simulink model "Mcl_Floating_Signal_Processing"  (R2018a)
settings: Solver=VariableStepAuto  StartTime=0.0  StopTime=10.0  RelTol=1e-3
libraries: mciapi_libbrowser x4
settings Model: Creator=lab.motori2  LastModifiedBy=lab.motori2

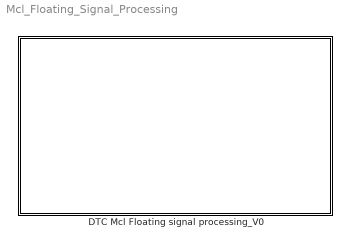
== system Mcl_Floating_Signal_Processing ==
  DTC Mcl Floating signal processing_V0 : Subsystem

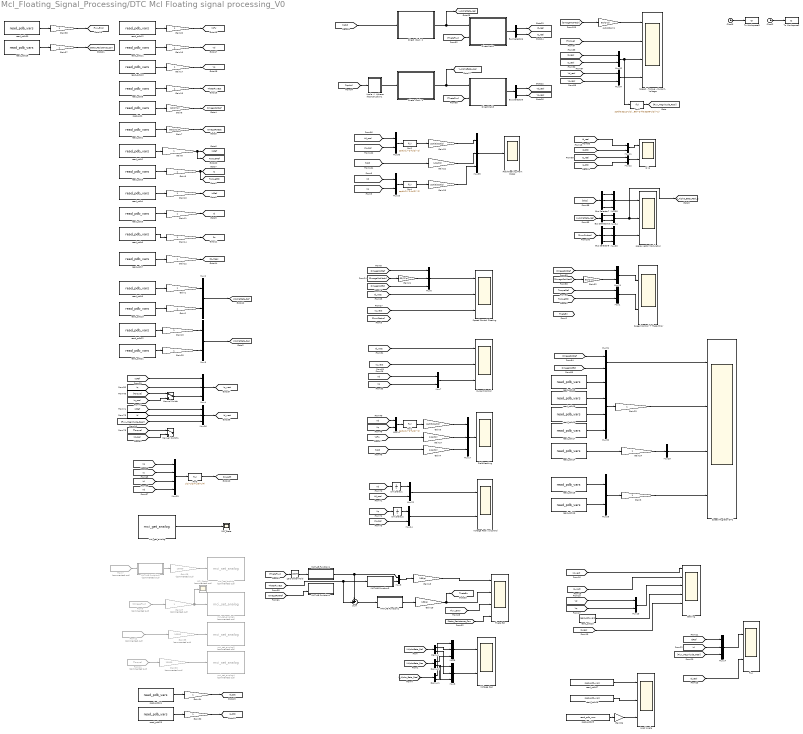
== system Mcl_Floating_Signal_Processing/DTC Mcl Floating signal processing_V0 ==
  Braking : Scope  NumInputPorts=6
  Bus Selector10 : BusSelector  OutputSignals=Alpha,Beta
  Bus Selector6 : BusSelector  OutputSignals=D,Q
  Bus Selector7 : BusSelector  OutputSignals=Ia,Ib,Ic
  Bus Selector8 : BusSelector  OutputSignals=A,B,C
  Bus Selector9 : BusSelector  OutputSignals=D,Q
  Clock2 : Clock
  Clock3 : Clock
  Current Control : Scope  NumInputPorts=3
  Demux : Demux  Outputs=2
  Demux1 : Demux  Outputs=2
  Demux2 : Demux  Outputs=2
  Direct  Clark  2 : MATLAB Function  TreatAsAtomicUnit=on  SystemSampleTime=SystemSampleTime  mask{SystemSampleTime=-1}
      mask prompts: SystemSampleTime "Simulink:blkprm_prompts:AllBlksSampleTime"
  Direct  Clark  3 : MATLAB Function  TreatAsAtomicUnit=on  SystemSampleTime=SystemSampleTime  mask{SystemSampleTime=-1}
      mask prompts: SystemSampleTime "Simulink:blkprm_prompts:AllBlksSampleTime"
  Direct Park2 : MATLAB Function  TreatAsAtomicUnit=on  SystemSampleTime=SystemSampleTime  mask{SystemSampleTime=-1}
      mask prompts: SystemSampleTime "Simulink:blkprm_prompts:AllBlksSampleTime"
  Direct Park3 : MATLAB Function  TreatAsAtomicUnit=on  SystemSampleTime=SystemSampleTime  mask{SystemSampleTime=-1}
      mask prompts: SystemSampleTime "Simulink:blkprm_prompts:AllBlksSampleTime"
  Fcn1 : Fcn  Expr=sqrt(u(1)^2+u(2)^2)
  Fcn2 : Fcn  Expr=sqrt(u(1)^2+u(2)^2)
  Fcn3 : Fcn  Expr=u(1)*u(2)+u(3)*u(4)
  Fcn4 : Fcn  Expr=sqrt(u(1)^2+u(2)^2)
  Fcn5 : Fcn  Expr=sqrt((0.0212*u(1)+0.0688)^2+(0.0299*u(2))^2)
  "FieldWeaking " : Scope
  FieldWeaking From Model : Scope
  Flux : Scope  NumInputPorts=2
  From11 : From  Commented=on  GotoTag=Torque  TagVisibility=global
  From12 : From  Commented=on  GotoTag=Flux_Magnitude_Real
  From7 : From  Commented=on  GotoTag=Stator_Flux_Position_Real
  From9 : From  Commented=on  GotoTag=OmegaFlux  TagVisibility=global
  Gain{1..3,8..17,20,23..25,30,34,37..38} (21 alike) : Gain  OutDataTypeStr=double  RndMeth=Zero
  Gain18 : Gain  Gain=180/pi
  Gain19 : Gain  Gain=180/pi
  Gain21 : Gain  Gain=60/(2*pi)  RndMeth=Round
  Gain22 : Gain  Gain=1/sqrt(2)
  Gain26 : Gain  Gain=sqrt(3)/sqrt(2)
  Gain27 : Gain  Gain=1/sqrt(2)
  Gain28 : Gain  Commented=on  Gain=10000  OutDataTypeStr=int32
  Gain29 : Gain  Commented=on  OutDataTypeStr=int32
  Gain31 : Gain  Gain=sqrt(3)/sqrt(2)
  Gain32 : Gain  Gain=60/(2*pi)  RndMeth=Round
  Gain33 : Gain  Commented=on  Gain=10000  OutDataTypeStr=int32
  Gain35 : Gain  Commented=on  Gain=10000  OutDataTypeStr=int32
  Gain36 : Gain  Gain=180/pi
  Gain4 : Gain  Gain=1/sqrt(2)
  Gain5 : Gain  Gain=sqrt(3)/sqrt(2)
  Gain6 : Gain  Gain=60/(2*pi)  OutDataTypeStr=double  RndMeth=Zero
  Gain7 : Gain  Gain=60/(2*pi)/4  OutDataTypeStr=double  RndMeth=Zero
  Id iq : Scope  NumInputPorts=2
  Load Angle : Scope  NumInputPorts=3
  MATLAB Function1 : MATLAB Function  TreatAsAtomicUnit=on
  MATLAB Function2 : MATLAB Function  TreatAsAtomicUnit=on
  MATLAB Function3 : MATLAB Function  TreatAsAtomicUnit=on
  MATLAB Function4 : MATLAB Function  TreatAsAtomicUnit=on
  MATLAB Function5 : MATLAB Function  Commented=on  TreatAsAtomicUnit=on
  MCI_State : Scope
  MCI_State1 : Scope  Commented=on
  Manual Switch : ManualSwitch
  Manual Switch1 : ManualSwitch
  Mux{1..3,7,9..13,18,21..22,24,28,31..32,34,36..37} (19 alike) : Mux  Inputs=2
  Mux{4..6,8,14,17,26,33,35,38} (10 alike) : Mux  Inputs=3
  Mux23 : Mux
  Mux29 : Mux  Inputs=1
  Mux30 : Mux
  Speed - Torque - Current - Voltage : Scope  NumInputPorts=4
  Speed Control + Theta Error : Scope  NumInputPorts=2
  "Speed Control Floating " : Scope  NumInputPorts=3
  "Speed Ruglator DTC " : Scope  NumInputPorts=4
  Sum : Sum  Inputs=+-|
  Theta Est : Scope  NumInputPorts=4
  To Workspace2 : ToWorkspace  VariableName=t2  SampleTime=-1
      settings: Save2DSignal=2-D array (concatenate along first dimension)
  To Workspace3 : ToWorkspace  VariableName=t3  SampleTime=-1
      settings: Save2DSignal=2-D array (concatenate along first dimension)
  Unit Delay1 : UnitDelay  SampleTime=-1
  Unit Delay2 : UnitDelay  SampleTime=-1
  Voltage Real vs Control : Scope  NumInputPorts=2
  Voltage Rec : Scope  NumInputPorts=2
  "Vpole -> Vphase reconstruction1" : MATLAB Function  TreatAsAtomicUnit=on
  Zero-Order Hold : ZeroOrderHold  SampleTime=0.000125
  mci_get_analog : S-Function  FunctionName=mci_get_analog  Parameters=read_data, choose_read_data  SFunctionDeploymentMode=off  EnableBusSupport=off  mask{choose_read_data=MCI_AI_INTERNAL_MCI_STATE, read_data=24}
      mask prompts: choose_read_data "Data to read"
      mask TypeOptions choose_read_data: MCI_AI_TARGET_SPEED_RPM_S16 | MCI_AI_SPEED_REFERENCE_RPM_S16 | MCI_AI_ACTUAL_SPEED_S16 | MCI_AI_SPEED_ERROR_RPM_S16 | MCI_AI_MEAN_SPEED_S16 | MCI_AI_RMS_MOTOR_CURRENT_S16 | MCI_AI_ACTIVE_POWER_S16 | MCI_AI_SHAFT_POWER_S16 | MCI_AI_MOTOR_TEMP_S16 | MCI_AI_STATOR_TEMP_S16 | MCI_AI_LOAD_TORQUE_S16 | MCI_AI_SHAFT_POSITION_DEG_S16 | MCI_AI_BUS_CURRENT_S16 | MCI_AI_BUS_VOLTAGE_S16 | MCI_AI_INVERTER_TEMP_S16 | MCI_AI_INVERTER_TEMP_RAW_DATA | MCI_AI_VOLTAGE_PHASE_A_S16 | MCI_AI_VOLTAGE_PHASE_B_S16 | MCI_AI_VOLTAGE_PHASE_C_S16 | MCI_AI_SPEED_LOOP_GAIN_TABLE_INDEX | MCI_AI_CURR_PHASE_A_S16 | MCI_AI_CURR_PHASE_B_S16 | MCI_AI_CURR_PHASE_C_S16 | MCI_AI_STATOR_RESISTANCE_S16 | MCI_AI_INTERNAL_MCI_STATE
      mask Callback read_data:
      | rd = get_param(gcb,'choose_read_data');
      | poenum = strcat('MCI_AI_TYPE.',rd);
      | i_32 = eval(['int32(' poenum ')']);
      | set_param(gcb,'read_data',int2str(i_32));
      mask Display:
      | disp = regexp(choose_read_data, 'MCI_AI_', 'split');
      | port_label('output', 1, disp{2});
  mci_set_analog : mciapi_libbrowser/mci_set_analog  Commented=on  choose_write_data=MCI_AO_SPEED_LOOP_PROP_GAIN_S16  write_data=0
      settings: SourceProductName=Sim Arch
  mci_set_analog1 : mciapi_libbrowser/mci_set_analog  Commented=on  choose_write_data=MCI_AO_SPEED_LOOP_INT_GAIN_S16  write_data=1
      settings: SourceProductName=Sim Arch
  mci_set_analog3 : mciapi_libbrowser/mci_set_analog  Commented=on  choose_write_data=MCI_AO_SOFTSTART_COUNTER_INDEX  write_data=4
      settings: SourceProductName=Sim Arch
  mci_set_analog4 : mciapi_libbrowser/mci_set_analog  Commented=on  choose_write_data=MCI_AO_SPEED_FIR_TAPS_TABLE_INDEX  write_data=3
      settings: SourceProductName=Sim Arch
  rad/s2Rpm1 : Gain  Gain=60/(2*pi)
  read_pdb : S-Function  FunctionName=read_pdb_vars  Parameters=vstring  SFunctionDeploymentMode=off  EnableBusSupport=off  mask{vstring=Mcl_IO.Speed_Rot_Ref}
      mask prompts: vstring "Variable to read"
      mask Display:
      | disp = vstring;
      | port_label('output', 1, disp);
  read_pdb1 : S-Function  FunctionName=read_pdb_vars  Parameters=vstring  SFunctionDeploymentMode=off  EnableBusSupport=off  mask{vstring=Mcl_Quantities.Speed_Rot}
      mask prompts: vstring "Variable to read"
      mask Display:
      | disp = vstring;
      | port_label('output', 1, disp);
  read_pdb10 : S-Function  FunctionName=read_pdb_vars  Parameters=vstring  SFunctionDeploymentMode=off  EnableBusSupport=off  mask{vstring=Mcl_Quantities.Vs_DQ.Q}
      mask prompts: vstring "Variable to read"
      mask Display:
      | disp = vstring;
      | port_label('output', 1, disp);
  read_pdb11 : S-Function  FunctionName=read_pdb_vars  Parameters=vstring  SFunctionDeploymentMode=off  EnableBusSupport=off  mask{vstring=Mcl_Quantities.Vs_DQ.D}
      mask prompts: vstring "Variable to read"
      mask Display:
      | disp = vstring;
      | port_label('output', 1, disp);
  read_pdb12 : S-Function  FunctionName=read_pdb_vars  Parameters=vstring  SFunctionDeploymentMode=off  EnableBusSupport=off  mask{vstring=Mcl_Quantities.Vs_Max_Filt}
      mask prompts: vstring "Variable to read"
      mask Display:
      | disp = vstring;
      | port_label('output', 1, disp);
  read_pdb13 : S-Function  FunctionName=read_pdb_vars  Parameters=vstring  SFunctionDeploymentMode=off  EnableBusSupport=off  mask{vstring=Speed_Controller.Upper_Limit}
      mask prompts: vstring "Variable to read"
      mask Display:
      | disp = vstring;
      | port_label('output', 1, disp);
  read_pdb14 : S-Function  FunctionName=read_pdb_vars  Parameters=vstring  SFunctionDeploymentMode=off  EnableBusSupport=off  mask{vstring=Load_Angle_Limiter.Err}
      mask prompts: vstring "Variable to read"
      mask Display:
      | disp = vstring;
      | port_label('output', 1, disp);
  read_pdb15 : S-Function  FunctionName=read_pdb_vars  Parameters=vstring  SFunctionDeploymentMode=off  EnableBusSupport=off  mask{vstring=Load_Angle_Limiter.Upper_Limit}
      mask prompts: vstring "Variable to read"
      mask Display:
      | disp = vstring;
      | port_label('output', 1, disp);
  read_pdb16 : S-Function  FunctionName=read_pdb_vars  Parameters=vstring  SFunctionDeploymentMode=off  EnableBusSupport=off  mask{vstring=Load_Angle_Limiter.Out}
      mask prompts: vstring "Variable to read"
      mask Display:
      | disp = vstring;
      | port_label('output', 1, disp);
  read_pdb17 : S-Function  FunctionName=read_pdb_vars  Parameters=vstring  SFunctionDeploymentMode=off  EnableBusSupport=off  mask{vstring=Speed_Controller.Lower_Limit}
      mask prompts: vstring "Variable to read"
      mask Display:
      | disp = vstring;
      | port_label('output', 1, disp);
  read_pdb18 : S-Function  FunctionName=read_pdb_vars  Parameters=vstring  SFunctionDeploymentMode=off  EnableBusSupport=off  mask{vstring=Speed_Controller.Out}
      mask prompts: vstring "Variable to read"
      mask Display:
      | disp = vstring;
      | port_label('output', 1, disp);
  read_pdb19 : S-Function  FunctionName=read_pdb_vars  Parameters=vstring  SFunctionDeploymentMode=off  EnableBusSupport=off  mask{vstring=Mcl_Quantities.Vs_Alpha_Beta.Beta}
      mask prompts: vstring "Variable to read"
      mask Display:
      | disp = vstring;
      | port_label('output', 1, disp);
  read_pdb2 : S-Function  FunctionName=read_pdb_vars  Parameters=vstring  SFunctionDeploymentMode=off  EnableBusSupport=off  mask{vstring=Mcl_Quantities.Torque_Ref}
      mask prompts: vstring "Variable to read"
      mask Display:
      | disp = vstring;
      | port_label('output', 1, disp);
  read_pdb20 : S-Function  FunctionName=read_pdb_vars  Parameters=vstring  SFunctionDeploymentMode=off  EnableBusSupport=off  mask{vstring=Mcl_Quantities.Torque_Ref}
      mask prompts: vstring "Variable to read"
      mask Display:
      | disp = vstring;
      | port_label('output', 1, disp);
  read_pdb21 : S-Function  FunctionName=read_pdb_vars  Parameters=vstring  SFunctionDeploymentMode=off  EnableBusSupport=off  mask{vstring=Mcl_Quantities.Vs_Alpha_Beta_Rec.Beta}
      mask prompts: vstring "Variable to read"
      mask Display:
      | disp = vstring;
      | port_label('output', 1, disp);
  read_pdb22 : S-Function  FunctionName=read_pdb_vars  Parameters=vstring  SFunctionDeploymentMode=off  EnableBusSupport=off  mask{vstring=Mcl_Quantities.Vs_Alpha_Beta_Rec.Alpha}
      mask prompts: vstring "Variable to read"
      mask Display:
      | disp = vstring;
      | port_label('output', 1, disp);
  read_pdb23 : S-Function  FunctionName=read_pdb_vars  Parameters=vstring  SFunctionDeploymentMode=off  EnableBusSupport=off  mask{vstring=rotor_curr_iq}
      mask prompts: vstring "Variable to read"
      mask Display:
      | disp = vstring;
      | port_label('output', 1, disp);
  read_pdb24 : S-Function  FunctionName=read_pdb_vars  Parameters=vstring  SFunctionDeploymentMode=off  EnableBusSupport=off  mask{vstring=rotor_curr_id}
      mask prompts: vstring "Variable to read"
      mask Display:
      | disp = vstring;
      | port_label('output', 1, disp);
  read_pdb25 : S-Function  FunctionName=read_pdb_vars  Parameters=vstring  SFunctionDeploymentMode=off  EnableBusSupport=off  mask{vstring=Id_Braking}
      mask prompts: vstring "Variable to read"
      mask Display:
      | disp = vstring;
      | port_label('output', 1, disp);
  read_pdb26 : S-Function  FunctionName=read_pdb_vars  Parameters=vstring  SFunctionDeploymentMode=off  EnableBusSupport=off  mask{vstring=Stator_Resistance_Corr}
      mask prompts: vstring "Variable to read"
      mask Display:
      | disp = vstring;
      | port_label('output', 1, disp);
  read_pdb27 : S-Function  FunctionName=read_pdb_vars  Parameters=vstring  SFunctionDeploymentMode=off  EnableBusSupport=off  mask{vstring=Mcl_Quantities.Load_Angle_Sin_Cos.Sin}
      mask prompts: vstring "Variable to read"
      mask Display:
      | disp = vstring;
      | port_label('output', 1, disp);
  read_pdb28 : S-Function  FunctionName=read_pdb_vars  Parameters=vstring  SFunctionDeploymentMode=off  EnableBusSupport=off  mask{vstring=Mcl_Quantities.Load_Angle_Sin_Cos.Cos}
      mask prompts: vstring "Variable to read"
      mask Display:
      | disp = vstring;
      | port_label('output', 1, disp);
  read_pdb29 : S-Function  FunctionName=read_pdb_vars  Parameters=vstring  SFunctionDeploymentMode=off  EnableBusSupport=off  mask{vstring=Mcl_Quantities.Load_Angle}
      mask prompts: vstring "Variable to read"
      mask Display:
      | disp = vstring;
      | port_label('output', 1, disp);
  read_pdb3 : S-Function  FunctionName=read_pdb_vars  Parameters=vstring  SFunctionDeploymentMode=off  EnableBusSupport=off  mask{vstring=Mcl_Quantities.Torque}
      mask prompts: vstring "Variable to read"
      mask Display:
      | disp = vstring;
      | port_label('output', 1, disp);
  read_pdb30 : S-Function  FunctionName=read_pdb_vars  Parameters=vstring  SFunctionDeploymentMode=off  EnableBusSupport=off  mask{vstring=Flux_Error}
      mask prompts: vstring "Variable to read"
      mask Display:
      | disp = vstring;
      | port_label('output', 1, disp);
  read_pdb4 : S-Function  FunctionName=read_pdb_vars  Parameters=vstring  SFunctionDeploymentMode=off  EnableBusSupport=off  mask{vstring=Mcl_Quantities.Flux_Ref}
      mask prompts: vstring "Variable to read"
      mask Display:
      | disp = vstring;
      | port_label('output', 1, disp);
  read_pdb5 : S-Function  FunctionName=read_pdb_vars  Parameters=vstring  SFunctionDeploymentMode=off  EnableBusSupport=off  mask{vstring=Mcl_Quantities.Stator_Flux_Mag}
      mask prompts: vstring "Variable to read"
      mask Display:
      | disp = vstring;
      | port_label('output', 1, disp);
  read_pdb6 : S-Function  FunctionName=read_pdb_vars  Parameters=vstring  SFunctionDeploymentMode=off  EnableBusSupport=off  mask{vstring=Mcl_Quantities.Stator_Resistance}
      mask prompts: vstring "Variable to read"
      mask Display:
      | disp = vstring;
      | port_label('output', 1, disp);
  read_pdb7 : S-Function  FunctionName=read_pdb_vars  Parameters=vstring  SFunctionDeploymentMode=off  EnableBusSupport=off  mask{vstring=Estimated_Resistance}
      mask prompts: vstring "Variable to read"
      mask Display:
      | disp = vstring;
      | port_label('output', 1, disp);
  read_pdb8 : S-Function  FunctionName=read_pdb_vars  Parameters=vstring  SFunctionDeploymentMode=off  EnableBusSupport=off  mask{vstring=Mcl_Quantities.Rotor_Position}
      mask prompts: vstring "Variable to read"
      mask Display:
      | disp = vstring;
      | port_label('output', 1, disp);
  read_pdb9 : S-Function  FunctionName=read_pdb_vars  Parameters=vstring  SFunctionDeploymentMode=off  EnableBusSupport=off  mask{vstring=Mcl_Quantities.Vs_Alpha_Beta.Alpha}
      mask prompts: vstring "Variable to read"
      mask Display:
      | disp = vstring;
      | port_label('output', 1, disp);
  space vector Modulation : Scope  NumInputPorts=3
  tag scope: Flux_Error=global, I_AlphaBeta_real=global, Id=global, IdRef=global, Id_Est=global, Id_real=global, Id_vect=global, Iq=global, IqRef=global, Iq_Est=global, Iq_real=global, Iq_vect=global, OmegaRotEst=global, OmegaRotRef=global, PowerEl=global, Rs=global, Rs_Meas=global, Stator_Resistance_Corr=global, ThetaErr=global, ThetaFluxEst=global, TorqueEst=global, TorqueRef=global, VAlphaBeta_Rec=global, VAlphaBeta_Ref=global, V_AlphaBeta_real=global, V_Alpha_Beta_Real_s=global, Vd=global, Vd_real=global, Vq=global, Vq_real=global, VsFw=global
  wires:
  [OmegaRotMech] -> Gain21/1
  Mux6/1 -> "Speed Control Floating "/1  "Speed Reference - Real - Estimated"
  [OmegaRotRef] -> Mux6/1
  [Id_vect] -> "Speed Control Floating "/2  "D Reference [Current on FOC - Flux on DTC]"
  Mux7/1 -> Current Control/3  "Vdq"
  [Vd] -> Mux7/1
  [Vq] -> Mux7/2
  [ThetaFlux] -> Zero-Order Hold/1
  Mux9/1 -> Gain18/1
  MATLAB Function1/1(Theta_out) -> Sum/1, Mux9/1
  Gain18/1 -> Theta Est/1  "Theta Flux Vs Theta Est"
  Sum/1 -> MATLAB Function2/1(Theta_in)
  Gain19/1 -> [ThetaErr], Theta Est/2  "Theta Err [deg]"
  MATLAB Function2/1(Theta_out) -> Gain19/1
  Fcn1/1 -> Gain5/1
  Mux18/1 -> Fcn1/1
  [Vd] -> Mux18/1
  [Vq] -> Mux18/2
  [VsFw] -> Gain27/1
  Mux17/1 -> "FieldWeaking "/1  "Vs Motor - VsLimit - Vdc"
  Gain27/1 -> Mux17/2  "Vs Limit"
  [Vdc] -> Gain4/1
  [OmegaRotRef] -> MATLAB Function4/2(omega_rot_ref)
  Mux22/1 -> Voltage Real vs Control/1  "Vd Control vs Vd Real"
  Mux24/1 -> Voltage Real vs Control/2  "Vq Control vs Vq Real"
  [Vd] -> Unit Delay1/1
  [Vq_real] -> Mux24/2
  [Vq] -> Unit Delay2/1
  [Vd_real] -> Mux22/2
  Unit Delay1/1 -> Mux22/1
  Unit Delay2/1 -> Mux24/1
  [Iq_vect] -> "Speed Control Floating "/3  "Q Reference [Current on FOC - Torque on DTC]"
  MATLAB Function3/1(Theta_out) -> Mux9/2
  Gain4/1 -> Mux17/3  "Vdc"
  Gain5/1 -> Mux17/1  "Vs_Motor"
  Zero-Order Hold/1 -> MATLAB Function1/1(Theta_in)
  [ThetaFluxEst] -> Sum/2, MATLAB Function3/1(Theta_in)
  Gain21/1 -> Mux6/2  "Speed Real"
  [OmegaRotEst] -> Mux6/3
  read_pdb15/1 -> Mux28/1
  Mux28/1 -> Gain3/1  "Load Angle"
  read_pdb16/1 -> Mux28/2
  Gain24/1 -> Mux29/1
  Mux29/1 -> "Speed Ruglator DTC "/3
  Mux31/1 -> "Speed Ruglator DTC "/1  "Speed"
  Mux30/1 -> Gain23/1
  Gain23/1 -> "Speed Ruglator DTC "/2  "Torque"
  read_pdb14/1 -> Gain24/1
  [OmegaRotRef] -> Mux31/1
  [OmegaRotEst] -> Mux31/2
  Mux36/1 -> Fcn2/1
  Fcn2/1 -> Gain31/1
  Bus Selector6/1 -> [Id_real]  "<D>"
  [Vpole] -> "Vpole -> Vphase reconstruction1"/1(Vpole)
  Mux38/1 -> space vector Modulation/1  "Current A B C"
  [Vq_real] -> Mux37/2  "Vq"
  Gain22/1 -> Mux35/2  "Vdc"
  Bus Selector6/2 -> [Iq_real]  "<Q>"
  Bus Selector7/2 -> Mux38/2  "<Ib>"
  [Vd_real] -> Mux36/1  "Vd_real"
  "Vpole -> Vphase reconstruction1"/1(Vout) -> Direct  Clark  3/1(Xabc)
  [Vq_real] -> Mux36/2  "Vq_real"
  [ThetaFlux] -> Direct Park3/2(Theta)
  Gain31/1 -> Mux35/1  "Vs_Motor"
  Mux32/1 -> Fcn5/1, Speed - Torque - Current - Voltage/3
  Direct Park2/1(Xdq) -> Bus Selector6/1
  Clock2/1 -> To Workspace2/1
  [Iq_real] -> Mux32/2  "Iq"
  rad/s2Rpm1/1 -> Speed - Torque - Current - Voltage/1  "Speed"
  [PwmDuties] -> Bus Selector8/1
  Bus Selector7/1 -> Mux38/1  "<Ia>"
  Bus Selector7/3 -> Mux38/3  "<Ic>"
  Mux37/1 -> Speed - Torque - Current - Voltage/4
  Clock3/1 -> To Workspace3/1
  [Iabc] -> Direct  Clark  2/1(Xabc)
  [Iabc] -> Bus Selector7/1
  Bus Selector9/1 -> [Vd_real]  "<D>"
  [ThetaFlux] -> Direct Park2/2(Theta)
  Bus Selector8/3 -> Mux33/3  "<C>"
  [Torque] -> Speed - Torque - Current - Voltage/2  "Torque"
  [Id_real] -> Mux32/1  "Id"
  Bus Selector10/1 -> Mux34/1  "<Alpha>"
  Mux33/1 -> space vector Modulation/3  "Pwm Duties"
  [Vd_real] -> Mux37/1  "Vd"
  Bus Selector9/2 -> [Vq_real]  "<Q>"
  Bus Selector10/2 -> Mux34/2  "<Beta>"
  Mux34/1 -> [V_Alpha_Beta_Real_s], space vector Modulation/2  "V Alpha Beta"
  Bus Selector8/1 -> Mux33/1  "<A>"
  Bus Selector8/2 -> Mux33/2  "<B>"
  [V_AlphaBeta_real] -> Bus Selector10/1
  Mux35/1 -> FieldWeaking From Model/1
  Direct  Clark  3/1(XAlphaBeta) -> Direct Park3/1(XAlphaBeta), [V_AlphaBeta_real]  "Valpha_Beta_reconstructed"
  [Vdc] -> Gain22/1  "Vdc"
  Direct Park3/1(Xdq) -> Bus Selector9/1
  Direct  Clark  2/1(XAlphaBeta) -> [I_AlphaBeta_real], Direct Park2/1(XAlphaBeta)
  [OmegaRotMech] -> rad/s2Rpm1/1
  Gain8/1 -> [TorqueRef], [IqRef]
  read_pdb4/1 -> Gain10/1
  Gain11/1 -> [Id]
  Gain9/1 -> [TorqueEst], [Iq]
  read_pdb/1 -> Gain6/1
  Gain14/1 -> [Rs]
  read_pdb10/1 -> Gain17/1
  Gain20/1 -> [VsFw]
  read_pdb7/1 -> Gain12/1
  Gain12/1 -> [Rs_Meas]
  read_pdb8/1 -> Gain15/1
  Gain15/1 -> [ThetaFluxEst]
  Gain17/1 -> [Vq]  "Vq"
  Gain10/1 -> [IdRef]
  read_pdb3/1 -> Gain9/1
  read_pdb5/1 -> Gain11/1
  read_pdb2/1 -> Gain8/1
  read_pdb12/1 -> Gain20/1
  Gain6/1 -> [OmegaRotRef]
  read_pdb1/1 -> Gain7/1
  read_pdb6/1 -> Gain14/1
  Gain16/1 -> [Vd]  "Vd"
  read_pdb11/1 -> Gain16/1
  Gain7/1 -> [OmegaRotEst]
  read_pdb17/1 -> Mux30/4
  read_pdb20/1 -> Mux30/3
  read_pdb18/1 -> Mux30/2
  Gain3/1 -> "Speed Ruglator DTC "/4  "Load Angle"
  [Id_vect] -> Current Control/1  "D Reference [Current on FOC - Flux on DTC"
  [Iq_vect] -> Current Control/2  "Q Reference [Current on FOC - Torque on DTC]"
  [TorqueEst] -> Mux1/2
  [TorqueRef] -> Mux1/1
  Mux1/1 -> Speed Control + Theta Error/2  "Torque"
  [OmegaRotMech] -> Gain32/1
  Gain32/1 -> Mux21/2  "Motor Speed"
  [OmegaRotRef] -> Mux21/1  "Target Speed"
  Mux21/1 -> Speed Control + Theta Error/1
  read_pdb13/1 -> Mux30/1
  [Id] -> Mux26/2
  [Iq] -> Mux4/2
  [IqRef] -> Mux4/1
  [Torque] -> Manual Switch1/1
  [Iq_real] -> Manual Switch/2
  [Torque] -> Manual Switch/1
  Mux26/1 -> [Id_vect]  "Id"
  Manual Switch/1 -> Mux4/3
  [IdRef] -> Mux26/1
  [Vq] -> Mux23/1
  [Id_real] -> Manual Switch1/2
  Fcn3/1 -> [PowerEl]  "Power"
  mci_get_analog/1 -> MCI_State/1  "MCI_State"
  Mux23/1 -> Fcn3/1
  Mux4/1 -> [Iq_vect]  "Iq"
  [Vd] -> Mux23/4
  [Id] -> Mux23/3
  [Iq] -> Mux23/2
  read_pdb19/1 -> Gain2/1
  read_pdb9/1 -> Gain1/1
  Gain1/1 -> Mux2/1
  Gain2/1 -> Mux2/2
  Mux2/1 -> [VAlphaBeta_Ref]  "V Alpha Beta Ref"
  Mux3/1 -> [VAlphaBeta_Rec]  "V Alpha Beta Rec"
  read_pdb22/1 -> Gain13/1
  Gain13/1 -> Mux3/1
  Gain25/1 -> Mux3/2
  read_pdb21/1 -> Gain25/1
  [Vd] -> Mux10/1
  Mux10/1 -> Fcn4/1
  Fcn4/1 -> Gain26/1
  [Vq] -> Mux10/2
  Gain26/1 -> Mux35/3  "Vs Motor Ref"
  [VAlphaBeta_Ref] -> Demux/1
  Mux5/1 -> Voltage Rec/1  "VAlpha"
  Demux1/2 -> Mux8/1
  Demux1/1 -> Mux5/1
  [V_Alpha_Beta_Real_s] -> Demux1/1
  Mux8/1 -> Voltage Rec/2  "VBeta"
  Demux2/2 -> Mux8/3
  [VAlphaBeta_Rec] -> Demux2/1
  Demux/2 -> Mux8/2
  Demux/1 -> Mux5/2
  Demux2/1 -> Mux5/3
  From7/1 -> MATLAB Function5/1(Theta_in)
  From9/1 -> Gain29/1
  Gain28/1 -> mci_set_analog/1
  Gain29/1 -> MCI_State1/1, mci_set_analog1/1
  MATLAB Function5/1(Theta_out) -> Gain28/1
  Gain35/1 -> mci_set_analog3/1
  Gain33/1 -> mci_set_analog4/1
  From11/1 -> Gain33/1
  [Flux_Magnitude_Real] -> Mux26/3
  From12/1 -> Gain35/1
  read_pdb24/1 -> Gain34/1
  Gain34/1 -> [Id_Est]
  Gain30/1 -> [Iq_Est]
  read_pdb23/1 -> Gain30/1
  [Id_real] -> Mux11/1  "Id_rot"
  [Id_Est] -> Mux11/2
  Mux11/1 -> Id iq/1
  Mux12/1 -> Id iq/2
  [Iq_real] -> Mux12/1  "Iq_rot"
  [Iq_Est] -> Mux12/2
  Mux13/1 -> Braking/3  "Vdq"
  [Vd] -> Mux13/1
  [Vq] -> Mux13/2
  [Id_vect] -> Braking/1  "D Reference [Current on FOC - Flux on DTC"
  [Iq_vect] -> Braking/2  "Q Reference [Current on FOC - Torque on DTC]"
  read_pdb25/1 -> Braking/4  "Id_Braking"
  [Id_real] -> Braking/5  "id_real"
  read_pdb27/1 -> Load Angle/1  "sin"
  read_pdb28/1 -> Load Angle/2  "cos"
  read_pdb29/1 -> Gain36/1
  Gain36/1 -> Load Angle/3
  Fcn5/1 -> [Flux_Magnitude_Real]
  [IdRef] -> Mux14/1
  [Id] -> Mux14/2
  [Flux_Magnitude_Real] -> Mux14/3
  Mux14/1 -> Flux/1
  [Id_real] -> Flux/2
  Gain38/1 -> [Flux_Error]
  Gain37/1 -> [Stator_Resistance_Corr]
  read_pdb30/1 -> Gain38/1
  read_pdb26/1 -> Gain37/1
  [Flux_Error] -> Theta Est/3
  [Stator_Resistance_Corr] -> Theta Est/4

== matlab function Mcl_Floating_Signal_Processing/DTC Mcl Floating signal processing_V0/Direct  Clark  3 ==
  data: XAlphaBeta output Bus: XAlphaBetaBus; Xabc input Bus: XabcBus
function XAlphaBeta = DirectClark(Xabc)

XAlphaBeta.Alpha = Xabc.A;
XAlphaBeta.Beta =  sqrt(3)/3*(Xabc.A+2*Xabc.B);

== matlab function Mcl_Floating_Signal_Processing/DTC Mcl Floating signal processing_V0/Direct  Clark  2 ==
  data: XAlphaBeta output Bus: XAlphaBetaBus; Xabc input Bus: XabcBus
function XAlphaBeta = DirectClark(Xabc)

XAlphaBeta.Alpha = Xabc.A;
XAlphaBeta.Beta =  sqrt(3)/3*(Xabc.A+2*Xabc.B);

== matlab function Mcl_Floating_Signal_Processing/DTC Mcl Floating signal processing_V0/MATLAB Function1 ==
  data: Theta_in input; Theta_out output
function Theta_out = fcn(Theta_in)
%#codegen

if(Theta_in > pi)||(Theta_in < -pi)
    
    Resto_pi =  mod(Theta_in, pi);
    Resto_2pi =  mod(Theta_in, 2*pi);
    
    
    if(Resto_pi ~= Resto_2pi)
    Theta_out = -pi+Resto_pi;
    else
    Theta_out = Resto_pi;    
    end
 
else
    
    Theta_out = Theta_in;
    
end

== matlab function Mcl_Floating_Signal_Processing/DTC Mcl Floating signal processing_V0/MATLAB Function2 ==
  data: Theta_in input; Theta_out output
function Theta_out = fcn(Theta_in)
%#codegen

if(Theta_in > pi)||(Theta_in < -pi)
    
    Resto_pi =  mod(Theta_in, pi);
    Resto_2pi =  mod(Theta_in, 2*pi);
    
    
    if(Resto_pi ~= Resto_2pi)
    Theta_out = -pi+Resto_pi;
    else
    Theta_out = Resto_pi;    
    end
 
else
    
    Theta_out = Theta_in;
    
end

== matlab function Mcl_Floating_Signal_Processing/DTC Mcl Floating signal processing_V0/Direct Park2 ==
  data: XAlphaBeta input Bus: XAlphaBetaBus; Xdq output Bus: XdqBus; Theta input
function Xdq = DirectPark(XAlphaBeta,Theta)

Xdq.D  =  XAlphaBeta.Alpha*cos(Theta) + XAlphaBeta.Beta*sin(Theta);
Xdq.Q  = -XAlphaBeta.Alpha*sin(Theta) + XAlphaBeta.Beta*cos(Theta);

== matlab function Mcl_Floating_Signal_Processing/DTC Mcl Floating signal processing_V0/MATLAB Function4 ==
  data: Theta_in input; Theta_out output; omega_rot_ref input
function Theta_out = fcn(Theta_in, omega_rot_ref)
%#codegen
if (omega_rot_ref < 0)
    
    Theta_in = 240/180*pi-Theta_in; 
    if(Theta_in > pi)||(Theta_in < -pi)

        Resto_pi =  mod(Theta_in, pi);
        Resto_2pi =  mod(Theta_in, 2*pi);


        if(Resto_pi ~= Resto_2pi)
        Theta_out = -pi+Resto_pi;
        else
        Theta_out = Resto_pi;    
        end

    else

        Theta_out = Theta_in;

    end    
else
    Theta_out = Theta_in;
end

== matlab function Mcl_Floating_Signal_Processing/DTC Mcl Floating signal processing_V0/MATLAB Function5 ==
  data: Theta_in input; Theta_out output
function Theta_out = fcn(Theta_in)
%#codegen

if(Theta_in > pi)||(Theta_in < -pi)
    
    Resto_pi =  mod(Theta_in, pi);
    Resto_2pi =  mod(Theta_in, 2*pi);
    
    
    if(Resto_pi ~= Resto_2pi)
    Theta_out = -pi+Resto_pi;
    else
    Theta_out = Resto_pi;    
    end
 
else
    
    Theta_out = Theta_in;
    
end

== matlab function Mcl_Floating_Signal_Processing/DTC Mcl Floating signal processing_V0/Direct Park3 ==
  data: XAlphaBeta input Bus: XAlphaBetaBus; Xdq output Bus: XdqBus; Theta input
function Xdq = DirectPark(XAlphaBeta,Theta)

Xdq.D  =  XAlphaBeta.Alpha*cos(Theta) + XAlphaBeta.Beta*sin(Theta);
Xdq.Q  = -XAlphaBeta.Alpha*sin(Theta) + XAlphaBeta.Beta*cos(Theta);

== matlab function Mcl_Floating_Signal_Processing/DTC Mcl Floating signal processing_V0/Vpole -> Vphase reconstruction1 ==
  data: Vpole input Bus: XabcBus size=1; Vout output Bus: XabcBus
function Vout   = Vrec2(Vpole)

Va = Vpole.A;
Vb = Vpole.B;
Vc = Vpole.C;

Vn = (Va + Vb + Vc)/3;

Vphase.A = Va - Vn;
Vphase.B = Vb - Vn;
Vphase.C = Vc - Vn;

Vline.A = Va - Vb;  % Vab
Vline.B = Vb - Vc;  % Vbc
Vline.C = Vc - Va;  % Vca

Vout = Vphase;
end

== matlab function Mcl_Floating_Signal_Processing/DTC Mcl Floating signal processing_V0/MATLAB Function3 ==
  data: Theta_in input; Theta_out output
function Theta_out = fcn(Theta_in)
%#codegen

if(Theta_in > pi)||(Theta_in < -pi)
    
    Resto_pi =  mod(Theta_in, pi);
    Resto_2pi =  mod(Theta_in, 2*pi);
    
    
    if(Resto_pi ~= Resto_2pi)
    Theta_out = -pi+Resto_pi;
    else
    Theta_out = Resto_pi;    
    end
 
else
    
    Theta_out = Theta_in;
    
end
